simulink model "stathmos_diodivn_me_2_e3ipiretes"  (R2019b)
settings: Solver=VariableStepAuto  StartTime=0.0  StopTime=10.0  RelTol=1e-3
undefined symbols (not defined in the file or in its folder): m, n, STime, STime1, STime2, STime3, Time, Time1, Time2, Time3
settings Model: Creator=Εμμανουήλ  LastModifiedBy=Εμμανουήλ

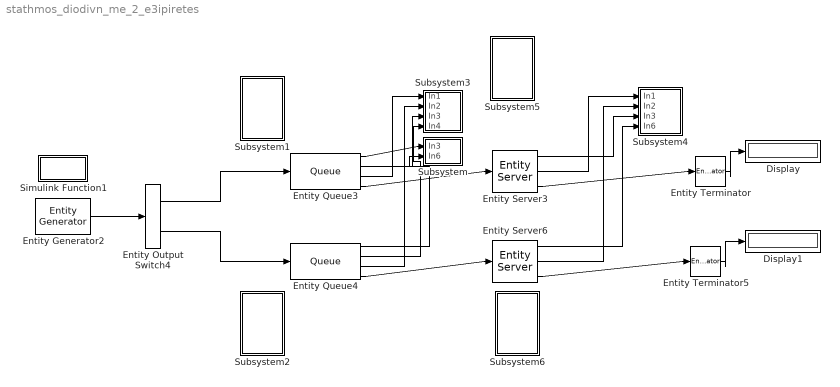
== system stathmos_diodivn_me_2_e3ipiretes ==
  Display : Display
      settings: Format=bank
  Display1 : Display
      settings: Format=bank
  Entity Output Switch4 : EntityOutputSwitch  InputPortMessageModes=m  OutputPortMessageModes=m,m  SwitchingCriterion=Equiprobable  SwitchAttributeName=Attribute1
  Entity Generator2 : EntityGenerator  OutputPortMessageModes=m  TimeSource=MATLAB action  IntergenerationTimeAction=dt=DT();  EntityType=Structured  EntityTypeName=Entity
  Entity Queue3 : Queue  InputPortMessageModes=m  OutputPortMessageModes=n,n,n,m  Capacity=inf  EntryAction=Time();  ExitAction=Time1();  NumberEntitiesInBlock=on  AverageWait=on  AverageQueueLength=on
      settings: OutputPortMap=o1,o2,o3,o5
  Entity Queue4 : Queue  InputPortMessageModes=m  OutputPortMessageModes=n,n,n,m  Capacity=inf  EntryAction=Time2();  ExitAction=Time3();  NumberEntitiesInBlock=on  AverageWait=on  AverageQueueLength=on
      settings: OutputPortMap=o1,o2,o3,o5
  Entity Server3 : EntityServer  InputPortMessageModes=m  OutputPortMessageModes=n,n,m  Capacity=1  ServiceTimeSource=MATLAB action  ServiceTimeAction=|  EntryAction=STime();  ExitAction=STime1();  AverageWait=on  Utilization=on
      | persistent rngInit;
      | if isempty(rngInit)
      |     seed = 12345;
      |     rng(seed);
      |     rngInit = true;
      | end
      | 
      | % Pattern: Gaussian (normal) distribution
      | % m: Mean, d: Standard deviation
      | m = 3; d = 4.5;
      | dt =120 + m + d * randn;
      settings: OutputPortMap=o4,o5,o9
  Entity Server6 : EntityServer  InputPortMessageModes=m  OutputPortMessageModes=n,n,m  Capacity=1  ServiceTimeSource=MATLAB action  ServiceTimeAction=|  EntryAction=STime2();  ExitAction=STime3();  AverageWait=on  Utilization=on
      | % Pattern: Gaussian (normal) distribution
      | % m: Mean, d: Standard deviation
      | m = 3; d = 4.5;
      | dt =120 + m + d * randn;
      settings: OutputPortMap=o4,o5,o9
  Entity Terminator : EntityTerminator  InputPortMessageModes=m  NumberEntitiesArrived=on
      settings: OutputPortMap=o0
  Entity Terminator5 : EntityTerminator  InputPortMessageModes=m  NumberEntitiesArrived=on
      settings: OutputPortMap=o0
  Simulink Function1 : Subsystem  TreatAsAtomicUnit=on
  Subsystem : Subsystem
  Subsystem1 : Subsystem
  Subsystem2 : Subsystem
  Subsystem3 : Subsystem
  Subsystem4 : Subsystem
  Subsystem5 : Subsystem
  Subsystem6 : Subsystem
  wires:
  Entity Queue3/2 -> Subsystem3/3(In3)
  Entity Queue4/3 -> Subsystem3/2(In2)
  Entity Queue4/2 -> Subsystem3/4(In4)
  Entity Queue3/3 -> Subsystem3/1(In1)
  Entity Server3/1 -> Subsystem4/3(In3)
  Entity Server6/1 -> Subsystem4/4(In6)
  Entity Generator2/1 -> Entity Output Switch4/1
  Entity Server6/2 -> Subsystem4/2(In2)
  Entity Output Switch4/1 -> Entity Queue3/1
  Entity Queue4/1 -> Subsystem/2(In6)
  Entity Terminator5/1 -> Display1/1
  Entity Server6/3 -> Entity Terminator5/1
  Entity Output Switch4/2 -> Entity Queue4/1
  Entity Terminator/1 -> Display/1
  Entity Queue3/1 -> Subsystem/1(In3)
  Entity Server3/2 -> Subsystem4/1(In1)
  Entity Queue4/4 -> Entity Server6/1
  Entity Queue3/4 -> Entity Server3/1
  Entity Server3/3 -> Entity Terminator/1

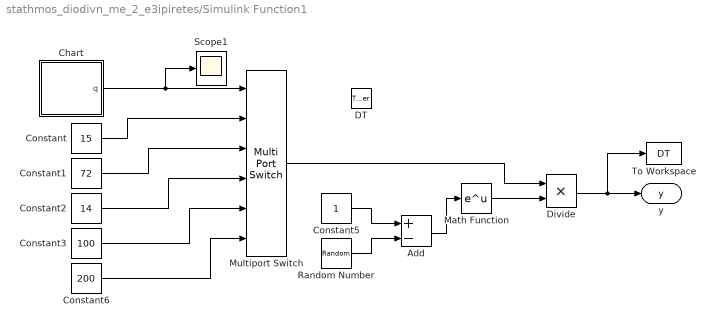
== system stathmos_diodivn_me_2_e3ipiretes/Simulink Function1 ==
  DT : TriggerPort  TriggerType=function-call  IsSimulinkFunction=on  FunctionName=DT  FunctionVisibility=scoped  VariantControl=(inherit)
  Add : Sum  Inputs=+-
  Chart : Stateflow chart  BlockKeywords=__PRM__SERIALIZED__DATA__:Stateflow Chart,Stateflow Diagram  TreatAsAtomicUnit=on
  Constant : Constant  Value=15
  Constant1 : Constant  Value=72
  Constant2 : Constant  Value=14
  Constant3 : Constant  Value=100
  Constant5 : Constant
  Constant6 : Constant  Value=200
  Divide : Product  Inputs=**
  Math Function : Math  SignedPower=off  SaturateOnIntegerOverflow=on
  Multiport Switch : MultiPortSwitch  DataPortOrder=Zero-based contiguous  Inputs=5  zeroidx=on
  Random Number : RandomNumber
  Scope1 : Scope
  To Workspace : ToWorkspace  VariableName=DT  SaveFormat=Timeseries  SampleTime=-1
      settings: Save2DSignal=2-D array (concatenate along first dimension)
  y : ArgOut  DisableCoverage=on  ArgumentName=y
  wires:
  Divide/1 -> To Workspace/1, y/1
  Add/1 -> Math Function/1
  Random Number/1 -> Add/2
  Constant5/1 -> Add/1
  Multiport Switch/1 -> Divide/1
  Math Function/1 -> Divide/2
  Constant3/1 -> Multiport Switch/5
  Constant2/1 -> Multiport Switch/4
  Constant1/1 -> Multiport Switch/3
  Constant/1 -> Multiport Switch/2
  Constant6/1 -> Multiport Switch/6
  Chart/1(q) -> Multiport Switch/1, Scope1/1

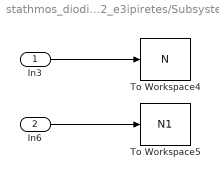
== system stathmos_diodivn_me_2_e3ipiretes/Subsystem ==
  In3 : Inport
  In6 : Inport  Port=2
  To Workspace4 : ToWorkspace  VariableName=N  SaveFormat=Timeseries  SampleTime=-1
      settings: Save2DSignal=2-D array (concatenate along first dimension)
  To Workspace5 : ToWorkspace  VariableName=N1  SaveFormat=Timeseries  SampleTime=-1
      settings: Save2DSignal=2-D array (concatenate along first dimension)
  wires:
  In3/1 -> To Workspace4/1
  In6/1 -> To Workspace5/1

== system stathmos_diodivn_me_2_e3ipiretes/Subsystem1 ==
  Simulink Function2 : Subsystem  TreatAsAtomicUnit=on
  Simulink Function3 : Subsystem  TreatAsAtomicUnit=on

== system stathmos_diodivn_me_2_e3ipiretes/Subsystem2 ==
  Simulink Function2 : Subsystem  TreatAsAtomicUnit=on
  Simulink Function3 : Subsystem  TreatAsAtomicUnit=on

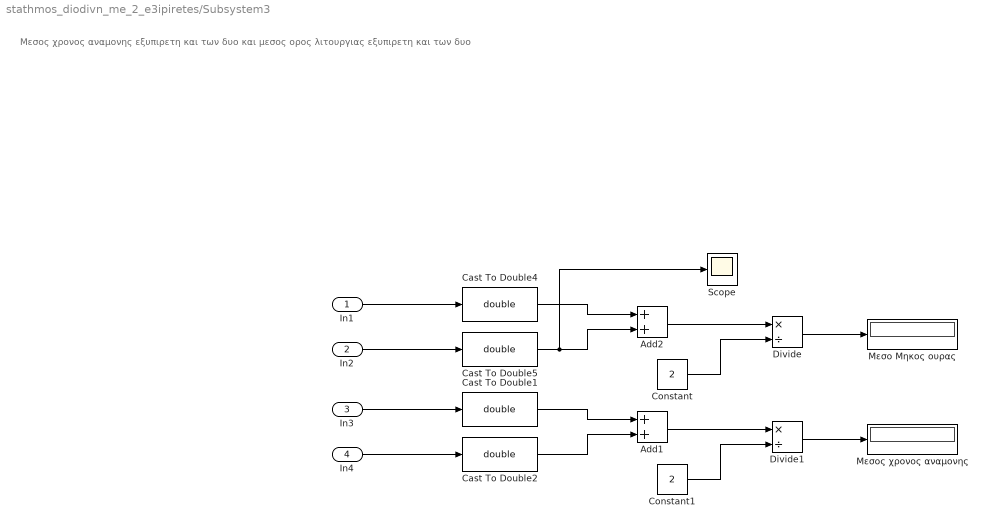
== system stathmos_diodivn_me_2_e3ipiretes/Subsystem3 ==
  note: Μεσος χρονος αναμονης εξυπιρετη και των δυο και μεσος ορος λιτουργιας εξυπιρετη και των δυο
  In1 : Inport
  In2 : Inport  Port=2
  In3 : Inport  Port=3
  In4 : Inport  Port=4
  Add1 : Sum
  Add2 : Sum
  Cast To Double{1..2,4..5} (4 alike) : DataTypeConversion  OutDataTypeStr=double
  Constant : Constant  Value=2
  Constant1 : Constant  Value=2
  Divide : Product  Inputs=*/
  Divide1 : Product  Inputs=*/
  Scope : Scope
  Μεσο Μηκος ουρας : Display
  Μεσος χρονος αναμονης : Display
  wires:
  In1/1 -> Cast To Double4/1
  Constant/1 -> Divide/2
  Divide/1 -> Μεσο Μηκος ουρας/1
  Cast To Double4/1 -> Add2/1
  Add2/1 -> Divide/1
  Add1/1 -> Divide1/1
  Cast To Double1/1 -> Add1/1
  Divide1/1 -> Μεσος χρονος αναμονης/1
  Constant1/1 -> Divide1/2
  Cast To Double2/1 -> Add1/2
  In4/1 -> Cast To Double2/1
  Cast To Double5/1 -> Scope/1, Add2/2
  In2/1 -> Cast To Double5/1
  In3/1 -> Cast To Double1/1

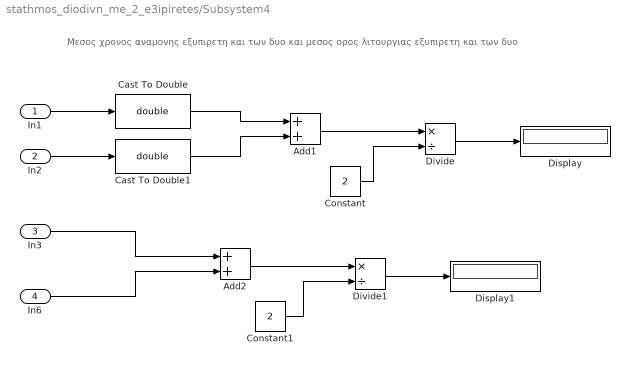
== system stathmos_diodivn_me_2_e3ipiretes/Subsystem4 ==
  note: Μεσος χρονος αναμονης εξυπιρετη και των δυο και μεσος ορος λιτουργιας εξυπιρετη και των δυο
  In1 : Inport
  In2 : Inport  Port=2
  In3 : Inport  Port=3
  In6 : Inport  Port=4
  Add1 : Sum
  Add2 : Sum
  Cast To Double : DataTypeConversion  OutDataTypeStr=double
  Cast To Double1 : DataTypeConversion  OutDataTypeStr=double
  Constant : Constant  Value=2
  Constant1 : Constant  Value=2
  Display : Display
  Display1 : Display
  Divide : Product  Inputs=*/
  Divide1 : Product  Inputs=*/
  wires:
  In6/1 -> Add2/2
  In3/1 -> Add2/1
  In1/1 -> Cast To Double/1
  In2/1 -> Cast To Double1/1
  Cast To Double/1 -> Add1/1
  Cast To Double1/1 -> Add1/2
  Add1/1 -> Divide/1
  Constant/1 -> Divide/2
  Divide/1 -> Display/1
  Divide1/1 -> Display1/1
  Constant1/1 -> Divide1/2
  Add2/1 -> Divide1/1

== system stathmos_diodivn_me_2_e3ipiretes/Subsystem5 ==
  Simulink Function2 : Subsystem  TreatAsAtomicUnit=on
  Simulink Function3 : Subsystem  TreatAsAtomicUnit=on

== system stathmos_diodivn_me_2_e3ipiretes/Subsystem6 ==
  Simulink Function2 : Subsystem  TreatAsAtomicUnit=on
  Simulink Function3 : Subsystem  TreatAsAtomicUnit=on

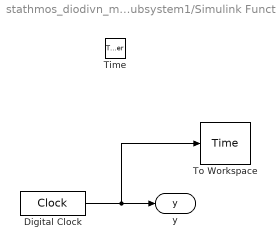
== system stathmos_diodivn_me_2_e3ipiretes/Subsystem1/Simulink Function2 ==
  Time : TriggerPort  TriggerType=function-call  IsSimulinkFunction=on  FunctionName=Time  VariantControl=(inherit)
  Digital Clock : DigitalClock  SampleTime=-1
  To Workspace : ToWorkspace  VariableName=Time  SampleTime=-1
      settings: Save2DSignal=2-D array (concatenate along first dimension)
  y : ArgOut  DisableCoverage=on  ArgumentName=y
  wires:
  Digital Clock/1 -> y/1, To Workspace/1

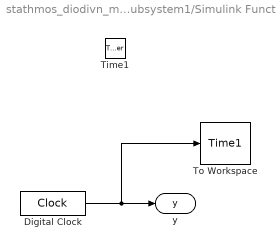
== system stathmos_diodivn_me_2_e3ipiretes/Subsystem1/Simulink Function3 ==
  Time1 : TriggerPort  TriggerType=function-call  IsSimulinkFunction=on  FunctionName=Time1  VariantControl=(inherit)
  Digital Clock : DigitalClock  SampleTime=-1
  To Workspace : ToWorkspace  VariableName=Time1  SampleTime=-1
      settings: Save2DSignal=2-D array (concatenate along first dimension)
  y : ArgOut  DisableCoverage=on  ArgumentName=y
  wires:
  Digital Clock/1 -> To Workspace/1, y/1

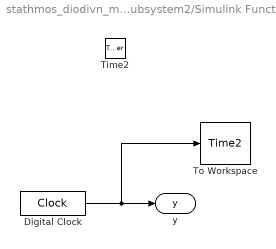
== system stathmos_diodivn_me_2_e3ipiretes/Subsystem2/Simulink Function2 ==
  Time2 : TriggerPort  TriggerType=function-call  IsSimulinkFunction=on  FunctionName=Time2  VariantControl=(inherit)
  Digital Clock : DigitalClock  SampleTime=-1
  To Workspace : ToWorkspace  VariableName=Time2  SampleTime=-1
      settings: Save2DSignal=2-D array (concatenate along first dimension)
  y : ArgOut  DisableCoverage=on  ArgumentName=y
  wires:
  Digital Clock/1 -> To Workspace/1, y/1

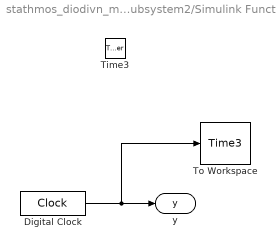
== system stathmos_diodivn_me_2_e3ipiretes/Subsystem2/Simulink Function3 ==
  Time3 : TriggerPort  TriggerType=function-call  IsSimulinkFunction=on  FunctionName=Time3  VariantControl=(inherit)
  Digital Clock : DigitalClock  SampleTime=-1
  To Workspace : ToWorkspace  VariableName=Time3  SampleTime=-1
      settings: Save2DSignal=2-D array (concatenate along first dimension)
  y : ArgOut  DisableCoverage=on  ArgumentName=y
  wires:
  Digital Clock/1 -> y/1, To Workspace/1

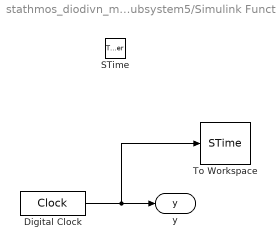
== system stathmos_diodivn_me_2_e3ipiretes/Subsystem5/Simulink Function2 ==
  STime : TriggerPort  TriggerType=function-call  IsSimulinkFunction=on  FunctionName=STime  VariantControl=(inherit)
  Digital Clock : DigitalClock  SampleTime=-1
  To Workspace : ToWorkspace  VariableName=STime  SampleTime=-1
      settings: Save2DSignal=2-D array (concatenate along first dimension)
  y : ArgOut  DisableCoverage=on  ArgumentName=y
  wires:
  Digital Clock/1 -> To Workspace/1, y/1

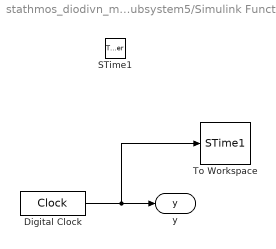
== system stathmos_diodivn_me_2_e3ipiretes/Subsystem5/Simulink Function3 ==
  STime1 : TriggerPort  TriggerType=function-call  IsSimulinkFunction=on  FunctionName=STime1  VariantControl=(inherit)
  Digital Clock : DigitalClock  SampleTime=-1
  To Workspace : ToWorkspace  VariableName=STime1  SampleTime=-1
      settings: Save2DSignal=2-D array (concatenate along first dimension)
  y : ArgOut  DisableCoverage=on  ArgumentName=y
  wires:
  Digital Clock/1 -> y/1, To Workspace/1

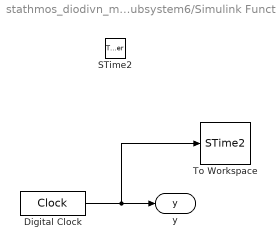
== system stathmos_diodivn_me_2_e3ipiretes/Subsystem6/Simulink Function2 ==
  STime2 : TriggerPort  TriggerType=function-call  IsSimulinkFunction=on  FunctionName=STime2  VariantControl=(inherit)
  Digital Clock : DigitalClock  SampleTime=-1
  To Workspace : ToWorkspace  VariableName=STime2  SampleTime=-1
      settings: Save2DSignal=2-D array (concatenate along first dimension)
  y : ArgOut  DisableCoverage=on  ArgumentName=y
  wires:
  Digital Clock/1 -> y/1, To Workspace/1

== system stathmos_diodivn_me_2_e3ipiretes/Subsystem6/Simulink Function3 ==
  STime3 : TriggerPort  TriggerType=function-call  IsSimulinkFunction=on  FunctionName=STime3  VariantControl=(inherit)
  Digital Clock : DigitalClock  SampleTime=-1
  To Workspace : ToWorkspace  VariableName=STime3  SampleTime=-1
      settings: Save2DSignal=2-D array (concatenate along first dimension)
  y : ArgOut  DisableCoverage=on  ArgumentName=y
  wires:
  Digital Clock/1 -> To Workspace/1, y/1

== stateflow chart stathmos_diodivn_me_2_e3ipiretes/Simulink Function1/Chart ==
  state wait_to_off1
    entry:q=4;
  state pump_off
    entry:q=0;
  state wait_to_off
    entry:q=3;
  state wait_to_on
    entry:q=1;
  state pump_on
    entry:q=2;
  wait_to_off -> wait_to_off1 : after(17280,sec)
  wait_to_off1 -> pump_off : after(17280,sec)
  (default) -> pump_off
  pump_off -> wait_to_on : after(17280,sec)
  pump_on -> wait_to_off : after(17280,sec)
  wait_to_on -> pump_on : after(17280,sec)
  data: q output
